simulink model "conSys_2robots_1_vR2014a"  (Simulink 8.3)
settings: Solver=FixedStepDiscrete  StartTime=0.0  StopTime=100  FixedStep=Ts  RelTol=1e-3
values from neighbouring files (symbols this model uses):
  ck = double(max(abs([par.q0_r1;par.q0_r2] - [par.q0r_r1;par.q0r_r2]))*20/7000 + 6)    [startUp_conSys_2robots_1_vGPU_vR2014a.m]    (also in startUp_conSys_2robots_1_vR2014a.m = max(abs([par.q0_r1;par.q0_r2] - [par.q0r_r1;par.q0r_r2]))*20; startUp_conSys_2robots_2_vR2014a.m = max(abs([par.q0_r1;par.q0_r2] - [par.q0r_r1;par.q0r_r2]))*20; startUp_conSys_2robots_3_vR2014a.m = max(abs([par.q0_r1;par.q0_r2] - [par.q0r_r1;par.q0r_r2]))*20; startUp_conSys_2robots_4_vR2014a.m = max(abs([par.q0_r1;par.q0_r2] - [par.q0r_r1;par.q0r_r2]))*20)
  d_0 = 2000    [startUp_conSys_2robots_1_vGPU_vR2014a.m]    (also in startUp_conSys_2robots_1_vR2014a.m = 200; startUp_conSys_2robots_2_vR2014a.m = 200; startUp_conSys_2robots_3_vR2014a.m; startUp_conSys_2robots_4_vR2014a.m = 200)
  do1r_0 = dthc_0 + dph1_0    (= 0.2)    [startUp_conSys_2robots_1_vGPU_vR2014a.m]    (also in startUp_conSys_2robots_1_vR2014a.m = 0; startUp_conSys_2robots_2_vR2014a.m = 0; startUp_conSys_2robots_3_vR2014a.m = 0; startUp_conSys_2robots_4_vR2014a.m = 0)
  do2r_0 = dthc_0 + dph2_0    (= -0.2)    [startUp_conSys_2robots_1_vGPU_vR2014a.m]    (also in startUp_conSys_2robots_1_vR2014a.m = 0; startUp_conSys_2robots_2_vR2014a.m = 0; startUp_conSys_2robots_3_vR2014a.m = 0; startUp_conSys_2robots_4_vR2014a.m = 0)
  dx1r_0 = dxc_0 + sin(thc_0)*dd_0 + d_0*cos(thc_0)*dthc_0    [startUp_conSys_2robots_1_vGPU_vR2014a.m]    (also in startUp_conSys_2robots_1_vR2014a.m; startUp_conSys_2robots_2_vR2014a.m; startUp_conSys_2robots_3_vR2014a.m; startUp_conSys_2robots_4_vR2014a.m)
  dx2r_0 = dxc_0 - sin(thc_0)*dd_0 - d_0*cos(thc_0)*dthc_0    [startUp_conSys_2robots_1_vGPU_vR2014a.m]    (also in startUp_conSys_2robots_1_vR2014a.m; startUp_conSys_2robots_2_vR2014a.m; startUp_conSys_2robots_3_vR2014a.m; startUp_conSys_2robots_4_vR2014a.m)
  dy1r_0 = dyc_0 + cos(thc_0)*dd_0 - d_0*sin(thc_0)*dthc_0    [startUp_conSys_2robots_1_vGPU_vR2014a.m]    (also in startUp_conSys_2robots_1_vR2014a.m; startUp_conSys_2robots_2_vR2014a.m; startUp_conSys_2robots_3_vR2014a.m; startUp_conSys_2robots_4_vR2014a.m)
  dy2r_0 = dyc_0 - cos(thc_0)*dd_0 + d_0*sin(thc_0)*dthc_0    [startUp_conSys_2robots_1_vGPU_vR2014a.m]    (also in startUp_conSys_2robots_1_vR2014a.m; startUp_conSys_2robots_2_vR2014a.m; startUp_conSys_2robots_3_vR2014a.m; startUp_conSys_2robots_4_vR2014a.m)
  o1r_0 = pi/2 - thc_0    (= 0)    [startUp_conSys_2robots_1_vGPU_vR2014a.m]    (also in startUp_conSys_2robots_1_vR2014a.m = pi/2 - thc_0; startUp_conSys_2robots_2_vR2014a.m = pi/2 - thc_0; startUp_conSys_2robots_3_vR2014a.m; startUp_conSys_2robots_4_vR2014a.m = th1_0)
  o2r_0 = pi/2 - thc_0    (= 0)    [startUp_conSys_2robots_1_vGPU_vR2014a.m]    (also in startUp_conSys_2robots_1_vR2014a.m = pi/2 - thc_0; startUp_conSys_2robots_2_vR2014a.m = pi/2 - thc_0; startUp_conSys_2robots_3_vR2014a.m; startUp_conSys_2robots_4_vR2014a.m = th2_0)
  thc_0 = pi/2    (= 1.57079632679)    [startUp_conSys_2robots_1_vGPU_vR2014a.m]    (also in startUp_conSys_2robots_1_vR2014a.m = atan2(1/25,1/12.5) + pi/2; startUp_conSys_2robots_2_vR2014a.m = atan2(1/25,1/12.5) + pi/2; startUp_conSys_2robots_3_vR2014a.m; startUp_conSys_2robots_4_vR2014a.m = atan2(1/25,1/12.5) + pi/2)
  Ts = 1/200    (= 0.005)    [startUp_conSys_2robots_1_vGPU_vR2014a.m]    (also in startUp_conSys_2robots_1_vR2014a.m = 0.0125; startUp_conSys_2robots_2_vR2014a.m = 0.01; startUp_conSys_2robots_3_vR2014a.m; startUp_conSys_2robots_4_vR2014a.m)
  x1_0 = 12000    [startUp_conSys_2robots_1_vGPU_vR2014a.m]    (also in startUp_conSys_2robots_1_vR2014a.m = 13178.9; startUp_conSys_2robots_2_vR2014a.m = 13178.9; startUp_conSys_2robots_3_vR2014a.m; startUp_conSys_2robots_4_vR2014a.m = 13178.9)
  x2_0 = 8000    [startUp_conSys_2robots_1_vGPU_vR2014a.m]    (also in startUp_conSys_2robots_1_vR2014a.m = 12821.1; startUp_conSys_2robots_2_vR2014a.m = 12821.1; startUp_conSys_2robots_3_vR2014a.m; startUp_conSys_2robots_4_vR2014a.m = 12821.1)
  xc_0 = 10000    [startUp_conSys_2robots_1_vGPU_vR2014a.m]    (also in startUp_conSys_2robots_1_vR2014a.m = 13000; startUp_conSys_2robots_2_vR2014a.m = 13000; startUp_conSys_2robots_3_vR2014a.m; startUp_conSys_2robots_4_vR2014a.m = 13000)
  y1_0 = 10000    [startUp_conSys_2robots_1_vGPU_vR2014a.m]    (also in startUp_conSys_2robots_1_vR2014a.m = 12910.6; startUp_conSys_2robots_2_vR2014a.m = 12910.6; startUp_conSys_2robots_3_vR2014a.m; startUp_conSys_2robots_4_vR2014a.m = 12910.6)
  y2_0 = 10000    [startUp_conSys_2robots_1_vGPU_vR2014a.m]    (also in startUp_conSys_2robots_1_vR2014a.m = 13089.4; startUp_conSys_2robots_2_vR2014a.m = 13089.4; startUp_conSys_2robots_3_vR2014a.m; startUp_conSys_2robots_4_vR2014a.m = 13089.4)
  yc_0 = 10000    [startUp_conSys_2robots_1_vGPU_vR2014a.m]    (also in startUp_conSys_2robots_1_vR2014a.m = 13000; startUp_conSys_2robots_2_vR2014a.m = 13000; startUp_conSys_2robots_3_vR2014a.m; startUp_conSys_2robots_4_vR2014a.m = 13000)
undefined symbols (not defined in the file or in its folder): absoluteAngle01_vR2014a, absoluteAngle02_vR2014a, DiscIntNeverNeededParam
undefined symbols (not defined in the file): ADAMS_cwd, ADAMS_exec, ADAMS_host, ADAMS_init, ADAMS_inputs, ADAMS_outputs, ADAMS_prefix, ADAMS_static, ADAMS_sysdir
libraries: simulink x18, cstblocks x7
(part 1 of 2)
settings Model: Creator=baqumau  LastModifiedBy=Mauro
settings DataIOCC: SignalLoggingSaveFormat=Dataset
settings DebuggingCC: UnderspecifiedInitializationDetection=Simplified  StateNameClashWarn=none
settings GRTTargetCC: CombineOutputUpdateFcns=on  GRTInterface=off

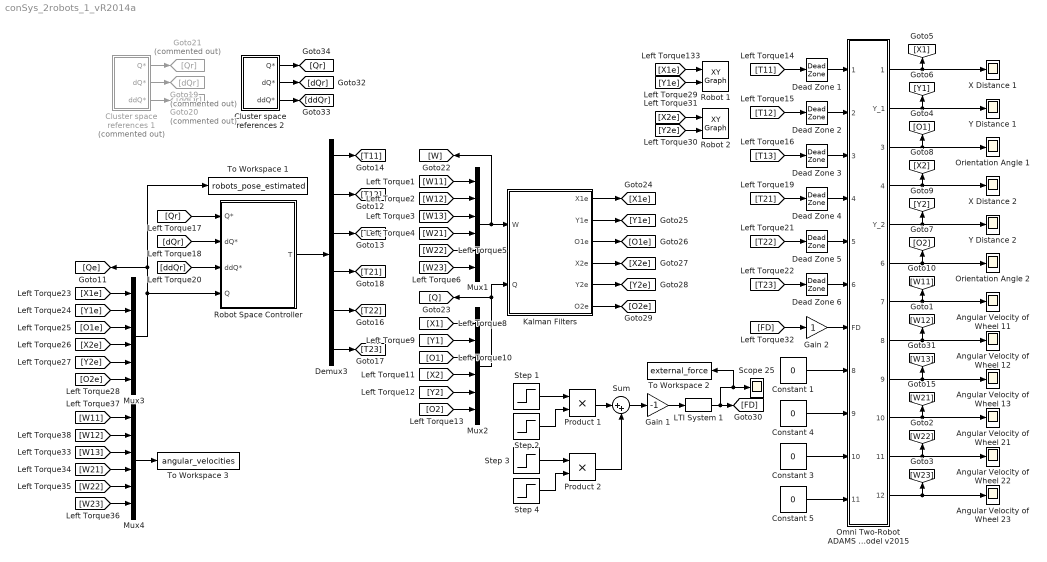
== system conSys_2robots_1_vR2014a ==
  Angular Velocity of Wheel {11..13,21..23} (6 alike) : Scope
      Angular Velocity of Wheel 11 settings: YMin=-1  YMax=20  SaveName=ScopeData3
      Angular Velocity of Wheel 12 settings: YMin=-1  YMax=20  SaveName=ScopeData6
      Angular Velocity of Wheel 13 settings: YMin=-1  YMax=1  SaveName=ScopeData9
      Angular Velocity of Wheel 21 settings: YMin=-1  YMax=1  SaveName=ScopeData2
      Angular Velocity of Wheel 22 settings: YMin=-1  YMax=1  SaveName=ScopeData10
      Angular Velocity of Wheel 23 settings: YMin=-1  YMax=1  SaveName=ScopeData11
  Cluster space references 1 : Subsystem  Commented=on
  Cluster space references 2 : Subsystem
  Constant {1,3..5} (4 alike) : Constant  Value=0
  Dead Zone {1..6} (6 alike) : DeadZone  LowerValue=-25  UpperValue=25  SaturateOnIntegerOverflow=on
  Demux3 : Demux  Outputs=6
  Gain 1 : Gain  Gain=-1
  Gain 2 : Gain
  Goto19 : Goto  Commented=on  GotoTag=dQr
  Goto20 : Goto  Commented=on  GotoTag=ddQr
  Goto21 : Goto  Commented=on  GotoTag=Qr
  Kalman Filters : Subsystem
  LTI System 1 : cstblocks/LTI System  sys=Fz  IC=[]
  Mux{1..4} (4 alike) : Mux  Inputs=6
  Omni Two-Robot ADAMS Model v2015 : Subsystem
  Orientation Angle 1 : Scope
      settings: YMin=-3  YMax=3
  Orientation Angle 2 : Scope
      settings: YMin=-3  YMax=3  SaveName=ScopeData12
  Product 1 : Product
  Product 2 : Product
  Robot 1 : simulink/Sinks/XY Graph  xmin=0  xmax=20000  ymin=0  ymax=20000  st=-1
  Robot 2 : simulink/Sinks/XY Graph  xmin=0  xmax=20000  ymin=0  ymax=20000  st=-1
  Robot Space Controller : Subsystem
  Scope 25 : Scope
      settings: YMin=-6  YMax=6  SaveName=ScopeData36
  Step 1 : Step  Time=60  SampleTime=0
  Step 2 : Step  Time=100  Before=1  After=0  SampleTime=0
  Step 3 : Step  Time=130  After=-1  SampleTime=0
  Step 4 : Step  Time=170  Before=1  After=0  SampleTime=0
  Sum : Sum  Inputs=|++
  To Workspace 1 : ToWorkspace  VariableName=robots_pose_estimated  SaveFormat=Structure With Time  SampleTime=-1
  To Workspace 2 : ToWorkspace  VariableName=external_force  SaveFormat=Structure With Time  SampleTime=-1
  To Workspace 3 : ToWorkspace  VariableName=angular_velocities  SaveFormat=Structure With Time  SampleTime=-1
  X Distance 1 : Scope
      settings: YMin=0  YMax=20000  SaveName=ScopeData4
  X Distance 2 : Scope
      settings: YMin=0  YMax=20000  SaveName=ScopeData16
  Y Distance 1 : Scope
      settings: YMin=0  YMax=20000
  Y Distance 2 : Scope
      settings: YMin=3000  YMax=3050  SaveName=ScopeData17
  wires:
  Omni Two-Robot ADAMS Model v2015/1(X_1) -> X Distance 1/1, [X1]
  Omni Two-Robot ADAMS Model v2015/2(Y_1) -> [Y1], Y Distance 1/1
  Omni Two-Robot ADAMS Model v2015/3(O_1) -> [O1], Orientation Angle 1/1
  Omni Two-Robot ADAMS Model v2015/7(W_11) -> [W11], Angular Velocity of Wheel 11/1
  Omni Two-Robot ADAMS Model v2015/10(W_21) -> [W21], Angular Velocity of Wheel 21/1
  Omni Two-Robot ADAMS Model v2015/9(W_13) -> Angular Velocity of Wheel 13/1, [W13]
  Omni Two-Robot ADAMS Model v2015/4(X_2) -> X Distance 2/1, [X2]
  Omni Two-Robot ADAMS Model v2015/5(Y_2) -> Y Distance 2/1, [Y2]
  Omni Two-Robot ADAMS Model v2015/6(O_2) -> Orientation Angle 2/1, [O2]
  Omni Two-Robot ADAMS Model v2015/8(W_12) -> Angular Velocity of Wheel 12/1, [W12]
  Omni Two-Robot ADAMS Model v2015/11(W_22) -> Angular Velocity of Wheel 22/1, [W22]
  Omni Two-Robot ADAMS Model v2015/12(W_23) -> [W23], Angular Velocity of Wheel 23/1
  [O1e] -> Mux3/3
  [X2e] -> Mux3/4
  [Y2e] -> Mux3/5
  [O2e] -> Mux3/6
  [X1e] -> Mux3/1
  [Y1e] -> Mux3/2
  [Qr] -> Robot Space Controller/1(Q*)
  [dQr] -> Robot Space Controller/2(dQ*)
  Mux3/1 -> Robot Space Controller/4(Q), [Qe], To Workspace 1/1
  Robot Space Controller/1(T) -> Demux3/1
  Demux3/1 -> [T11]
  Demux3/2 -> [T12]
  Demux3/3 -> [T13]
  Demux3/4 -> [T21]
  Demux3/5 -> [T22]
  Demux3/6 -> [T23]
  Cluster space references 1/1(Q*) -> Goto21/1
  Cluster space references 1/2(dQ*) -> Goto19/1
  Cluster space references 1/3(ddQ*) -> Goto20/1
  [ddQr] -> Robot Space Controller/3(ddQ*)
  [W13] -> Mux1/3
  [W21] -> Mux1/4
  [W22] -> Mux1/5
  [W23] -> Mux1/6
  [W11] -> Mux1/1
  [W12] -> Mux1/2
  Mux1/1 -> Kalman Filters/1(W), [W]
  [O1] -> Mux2/3
  [X2] -> Mux2/4
  [Y2] -> Mux2/5
  [O2] -> Mux2/6
  [X1] -> Mux2/1
  [Y1] -> Mux2/2
  Mux2/1 -> Kalman Filters/2(Q), [Q]
  Kalman Filters/1(X1e) -> [X1e]
  Kalman Filters/2(Y1e) -> [Y1e]
  Kalman Filters/3(O1e) -> [O1e]
  Kalman Filters/4(X2e) -> [X2e]
  Kalman Filters/5(Y2e) -> [Y2e]
  Kalman Filters/6(O2e) -> [O2e]
  [T11] -> Dead Zone 1/1
  [T12] -> Dead Zone 2/1
  [T13] -> Dead Zone 3/1
  [T21] -> Dead Zone 4/1
  [T22] -> Dead Zone 5/1
  [T23] -> Dead Zone 6/1
  [FD] -> Gain 2/1
  Constant 1/1 -> Omni Two-Robot ADAMS Model v2015/8(FX_1)
  Constant 3/1 -> Omni Two-Robot ADAMS Model v2015/10(FY_1)
  Constant 4/1 -> Omni Two-Robot ADAMS Model v2015/9(FX_2)
  Constant 5/1 -> Omni Two-Robot ADAMS Model v2015/11(FY_2)
  [X1e] -> Robot 1/1
  [Y1e] -> Robot 1/2
  [X2e] -> Robot 2/1
  [Y2e] -> Robot 2/2
  Step 1/1 -> Product 1/1
  Step 2/1 -> Product 1/2
  Step 3/1 -> Product 2/1
  Step 4/1 -> Product 2/2
  Product 1/1 -> Sum/1
  Product 2/1 -> Sum/2
  Sum/1 -> Gain 1/1
  LTI System 1/1 -> To Workspace 2/1, Scope 25/1, [FD]
  Gain 1/1 -> LTI System 1/1
  [W13] -> Mux4/3
  [W21] -> Mux4/4
  [W22] -> Mux4/5
  [W23] -> Mux4/6
  [W11] -> Mux4/1
  [W12] -> Mux4/2
  Mux4/1 -> To Workspace 3/1
  Gain 2/1 -> Omni Two-Robot ADAMS Model v2015/7(FD)
  Cluster space references 2/1(Q*) -> [Qr]
  Cluster space references 2/2(dQ*) -> [dQr]
  Cluster space references 2/3(ddQ*) -> [ddQr]
  Dead Zone 1/1 -> Omni Two-Robot ADAMS Model v2015/1(T_11)
  Dead Zone 2/1 -> Omni Two-Robot ADAMS Model v2015/2(T_12)
  Dead Zone 3/1 -> Omni Two-Robot ADAMS Model v2015/3(T_13)
  Dead Zone 4/1 -> Omni Two-Robot ADAMS Model v2015/4(T_21)
  Dead Zone 5/1 -> Omni Two-Robot ADAMS Model v2015/5(T_22)
  Dead Zone 6/1 -> Omni Two-Robot ADAMS Model v2015/6(T_23)

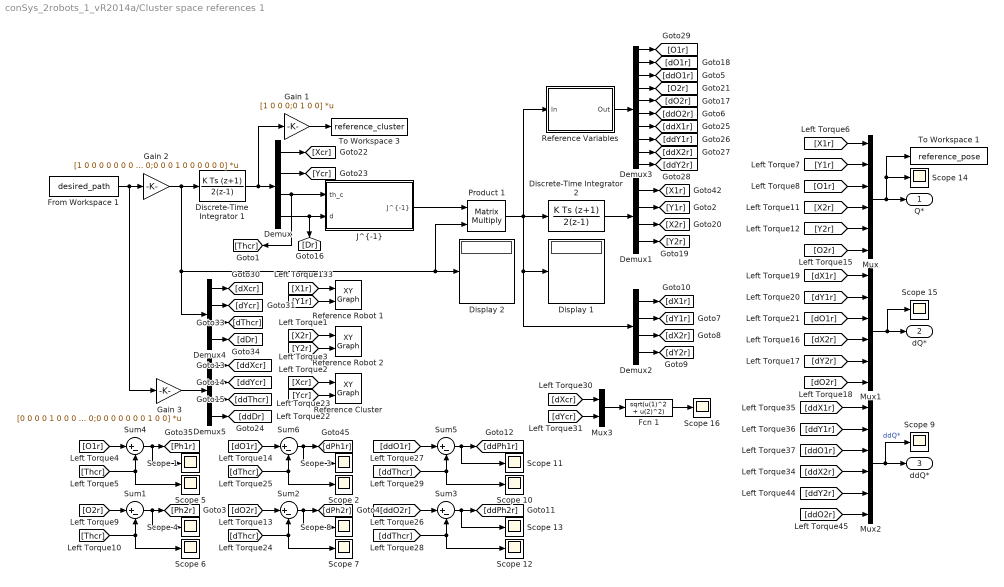
== system conSys_2robots_1_vR2014a/Cluster space references 1 ==
  Demux{,1..2,4..5} (5 alike) : Demux
  Demux3 : Demux  Outputs=10
  Discrete-Time Integrator 1 : DiscreteIntegrator  IntegratorMethod=Integration: Trapezoidal  InitialCondition=[xc_0 yc_0 thc_0 d_0]'  SampleTime=Ts  ICPrevOutput=DiscIntNeverNeededParam  ICPrevScaledInput=DiscIntNeverNeededParam
  Discrete-Time Integrator 2 : DiscreteIntegrator  IntegratorMethod=Integration: Trapezoidal  InitialCondition=[x1_0 y1_0 x2_0 y2_0]'  SampleTime=Ts  ICPrevOutput=DiscIntNeverNeededParam  ICPrevScaledInput=DiscIntNeverNeededParam
  Display 1 : Display
  Display 2 : Display
  Fcn 1 : Fcn  Expr=sqrt(u(1)^2 + u(2)^2)
  From Workspace 1 : FromWorkspace  VariableName=desired_path  SampleTime=Ts  OutputAfterFinalValue=Holding final value
  Gain 1 : Gain  Gain=[1 0 0 0;0 1 0 0]  Multiplication=Matrix(K*u)
  Gain 2 : Gain  Gain=[1 0 0 0 0 0 0 0 0 0;0 1 0 0 0 0 0 0 0 0;0 0 1 0 0 0 0 0 0 0;0 0 0 1 0 0 0 0 0 0]  Multiplication=Matrix(K*u)
  Gain 3 : Gain  Gain=[0 0 0 0 1 0 0 0 0 0;0 0 0 0 0 1 0 0 0 0;0 0 0 0 0 0 1 0 0 0;0 0 0 0 0 0 0 1 0 0]  Multiplication=Matrix(K*u)
  "J^{-1}" : Subsystem
  Mux : Mux  Inputs=6
  Mux1 : Mux  Inputs=6
  Mux2 : Mux  Inputs=6
  Mux3 : Mux  Inputs=2
  Product 1 : Product  Multiplication=Matrix(*)
  Reference Cluster : simulink/Sinks/XY Graph  xmin=0  xmax=20000  ymin=0  ymax=20000  st=-1
  Reference Robot 1 : simulink/Sinks/XY Graph  xmin=0  xmax=20000  ymin=0  ymax=20000  st=-1
  Reference Robot 2 : simulink/Sinks/XY Graph  xmin=0  xmax=20000  ymin=0  ymax=20000  st=-1
  Reference Variables : Subsystem
  Scope {1..16} (16 alike) : Scope
      Scope 1 settings: TimeRange=500  YMin=-15  YMax=15  SaveName=ScopeData52
      Scope 10 settings: TimeRange=500  YMin=-15  YMax=15  SaveName=ScopeData28
      Scope 11 settings: TimeRange=500  YMin=-15  YMax=15  SaveName=ScopeData42
      Scope 12 settings: TimeRange=500  YMin=-15  YMax=15  SaveName=ScopeData60
      Scope 13 settings: TimeRange=500  YMin=-15  YMax=15  SaveName=ScopeData66
      Scope 14 settings: ShowLegends=on  TimeRange=500  YMin=-6  YMax=0  SaveName=ScopeData59
      Scope 15 settings: ShowLegends=on  TimeRange=500  YMin=-1  YMax=1  SaveName=ScopeData69
      Scope 16 settings: ShowLegends=on  TimeRange=500  YMin=-50  YMax=200  SaveName=ScopeData18
      Scope 2 settings: TimeRange=500  YMin=-1  YMax=1  SaveName=ScopeData53
      Scope 3 settings: TimeRange=500  YMin=-1  YMax=1  SaveName=ScopeData79
      Scope 4 settings: TimeRange=500  YMin=-15  YMax=15  SaveName=ScopeData62
      Scope 5 settings: TimeRange=500  YMin=-15  YMax=15  SaveName=ScopeData81
      Scope 6 settings: TimeRange=500  YMin=-15  YMax=15  SaveName=ScopeData63
      Scope 7 settings: TimeRange=500  YMin=-15  YMax=15  SaveName=ScopeData64
      Scope 8 settings: TimeRange=500  YMin=-1  YMax=1  SaveName=ScopeData65
      Scope 9 settings: ShowLegends=on  TimeRange=500  YMin=-0.15  YMax=0.15  SaveName=ScopeData80
  Sum{1..6} (6 alike) : Sum  Inputs=|+-
  To Workspace 1 : ToWorkspace  VariableName=reference_pose  SaveFormat=Structure With Time  SampleTime=-1
  To Workspace 3 : ToWorkspace  VariableName=reference_cluster  SaveFormat=Structure With Time  SampleTime=-1
  Q* : Outport
  dQ* : Outport  Port=2
  ddQ* : Outport  Port=3
  wires:
  Demux4/1 -> [dXcr]
  Demux4/2 -> [dYcr]
  Demux4/4 -> [dDr]
  [Thcr] -> Scope 5/1, Sum4/2
  Demux4/3 -> [dThcr]
  Sum6/1 -> Scope 3/1, [dPh1r]
  Sum4/1 -> Scope 1/1, [Ph1r]
  [O1r] -> Sum4/1
  [dO1r] -> Sum6/1
  [dThcr] -> Scope 2/1, Sum6/2
  "J^{-1}"/1("J^{-1}") -> Product 1/1
  Product 1/1 -> Reference Variables/1(In), Demux2/1, Display 1/1, Discrete-Time Integrator 2/1
  [X1r] -> Reference Robot 1/1
  [Y1r] -> Reference Robot 1/2
  [X2r] -> Reference Robot 2/1
  [Y2r] -> Reference Robot 2/2
  From Workspace 1/1 -> Gain 3/1, Gain 2/1
  Discrete-Time Integrator 2/1 -> Demux1/1
  Demux1/1 -> [X1r]
  Demux1/2 -> [Y1r]
  Demux1/3 -> [X2r]
  Demux1/4 -> [Y2r]
  Reference Variables/1(Out) -> Demux3/1
  Demux3/1 -> [O1r]
  Demux3/2 -> [dO1r]
  Discrete-Time Integrator 1/1 -> Gain 1/1, Demux/1
  Demux/1 -> [Xcr]
  Demux/2 -> [Ycr]
  Demux/3 -> [Thcr], "J^{-1}"/1(th_c)
  Demux/4 -> [Dr], "J^{-1}"/2(d)
  Gain 1/1 -> To Workspace 3/1
  [X2r] -> Mux/4
  [O1r] -> Mux/3
  [Y1r] -> Mux/2
  [Y2r] -> Mux/5
  [X1r] -> Mux/1
  [O2r] -> Mux/6
  [dX2r] -> Mux1/4
  [dX1r] -> Mux1/1
  [dO1r] -> Mux1/3
  [dO2r] -> Mux1/6
  [dY2r] -> Mux1/5
  [dY1r] -> Mux1/2
  Mux/1 -> To Workspace 1/1, Scope 14/1, Q*/1
  Mux1/1 -> Scope 15/1, dQ*/1
  [Xcr] -> Reference Cluster/1
  [Ycr] -> Reference Cluster/2
  [Thcr] -> Sum1/2, Scope 6/1
  Sum1/1 -> [Ph2r], Scope 4/1
  [O2r] -> Sum1/1
  Sum2/1 -> [dPh2r], Scope 8/1
  [dO2r] -> Sum2/1
  [dThcr] -> Sum2/2, Scope 7/1
  Demux2/1 -> [dX1r]
  Demux2/2 -> [dY1r]
  Demux2/3 -> [dX2r]
  Demux2/4 -> [dY2r]
  Mux2/1 -> ddQ*/1, Scope 9/1  "ddQ*"
  [ddX1r] -> Mux2/1
  [ddY1r] -> Mux2/2
  [ddO1r] -> Mux2/3
  [ddX2r] -> Mux2/4
  [ddY2r] -> Mux2/5
  [ddO2r] -> Mux2/6
  Gain 2/1 -> Demux4/1, Product 1/2, Display 2/1, Discrete-Time Integrator 1/1
  Gain 3/1 -> Demux5/1
  Demux5/1 -> [ddXcr]
  Demux5/2 -> [ddYcr]
  Demux5/3 -> [ddThcr]
  Demux5/4 -> [ddDr]
  Demux3/4 -> [O2r]
  Demux3/5 -> [dO2r]
  Demux3/3 -> [ddO1r]
  Demux3/6 -> [ddO2r]
  Sum5/1 -> [ddPh1r], Scope 11/1
  [ddO1r] -> Sum5/1
  [ddThcr] -> Sum5/2, Scope 10/1
  Sum3/1 -> Scope 13/1, [ddPh2r]
  [ddO2r] -> Sum3/1
  [ddThcr] -> Scope 12/1, Sum3/2
  Demux3/7 -> [ddX1r]
  Demux3/8 -> [ddY1r]
  Demux3/9 -> [ddX2r]
  Demux3/10 -> [ddY2r]
  [dXcr] -> Mux3/1
  [dYcr] -> Mux3/2
  Mux3/1 -> Fcn 1/1
  Fcn 1/1 -> Scope 16/1

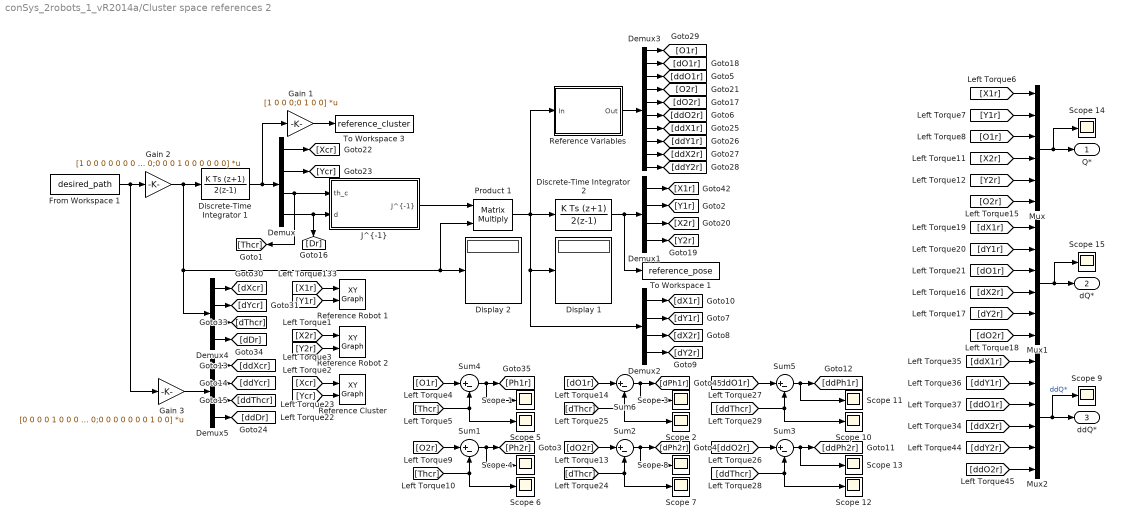
== system conSys_2robots_1_vR2014a/Cluster space references 2 ==
  Demux{,1..2,4..5} (5 alike) : Demux
  Demux3 : Demux  Outputs=10
  Discrete-Time Integrator 1 : DiscreteIntegrator  IntegratorMethod=Integration: Trapezoidal  InitialCondition=[xc_0 yc_0 thc_0 d_0]'  SampleTime=Ts  ICPrevOutput=DiscIntNeverNeededParam  ICPrevScaledInput=DiscIntNeverNeededParam
  Discrete-Time Integrator 2 : DiscreteIntegrator  IntegratorMethod=Integration: Trapezoidal  InitialCondition=[x1_0 y1_0 x2_0 y2_0]'  SampleTime=Ts  ICPrevOutput=DiscIntNeverNeededParam  ICPrevScaledInput=DiscIntNeverNeededParam
  Display 1 : Display
  Display 2 : Display
  From Workspace 1 : FromWorkspace  VariableName=desired_path  SampleTime=Ts  OutputAfterFinalValue=Holding final value
  Gain 1 : Gain  Gain=[1 0 0 0;0 1 0 0]  Multiplication=Matrix(K*u)
  Gain 2 : Gain  Gain=[1 0 0 0 0 0 0 0 0 0;0 1 0 0 0 0 0 0 0 0;0 0 1 0 0 0 0 0 0 0;0 0 0 1 0 0 0 0 0 0]  Multiplication=Matrix(K*u)
  Gain 3 : Gain  Gain=[0 0 0 0 1 0 0 0 0 0;0 0 0 0 0 1 0 0 0 0;0 0 0 0 0 0 1 0 0 0;0 0 0 0 0 0 0 1 0 0]  Multiplication=Matrix(K*u)
  "J^{-1}" : Subsystem
  Mux : Mux  Inputs=6
  Mux1 : Mux  Inputs=6
  Mux2 : Mux  Inputs=6
  Product 1 : Product  Multiplication=Matrix(*)
  Reference Cluster : simulink/Sinks/XY Graph  xmin=0  xmax=20000  ymin=0  ymax=20000  st=-1
  Reference Robot 1 : simulink/Sinks/XY Graph  xmin=0  xmax=20000  ymin=0  ymax=20000  st=-1
  Reference Robot 2 : simulink/Sinks/XY Graph  xmin=0  xmax=20000  ymin=0  ymax=20000  st=-1
  Reference Variables : Subsystem
  Scope {1..15} (15 alike) : Scope
      Scope 1 settings: TimeRange=500  YMin=-15  YMax=15  SaveName=ScopeData52
      Scope 10 settings: TimeRange=500  YMin=-15  YMax=15  SaveName=ScopeData28
      Scope 11 settings: TimeRange=500  YMin=-15  YMax=15  SaveName=ScopeData42
      Scope 12 settings: TimeRange=500  YMin=-15  YMax=15  SaveName=ScopeData60
      Scope 13 settings: TimeRange=500  YMin=-15  YMax=15  SaveName=ScopeData66
      Scope 14 settings: ShowLegends=on  TimeRange=500  YMin=-6  YMax=0  SaveName=ScopeData59
      Scope 15 settings: ShowLegends=on  TimeRange=500  YMin=-1  YMax=1  SaveName=ScopeData69
      Scope 2 settings: TimeRange=500  YMin=-15  YMax=15  SaveName=ScopeData53
      Scope 3 settings: TimeRange=500  YMin=-15  YMax=15  SaveName=ScopeData79
      Scope 4 settings: TimeRange=500  YMin=-15  YMax=15  SaveName=ScopeData62
      Scope 5 settings: TimeRange=500  YMin=-15  YMax=15  SaveName=ScopeData81
      Scope 6 settings: TimeRange=500  YMin=-15  YMax=15  SaveName=ScopeData63
      Scope 7 settings: TimeRange=500  YMin=-15  YMax=15  SaveName=ScopeData64
      Scope 8 settings: TimeRange=500  YMin=-15  YMax=15  SaveName=ScopeData65
      Scope 9 settings: ShowLegends=on  TimeRange=500  YMin=-0.15  YMax=0.15  SaveName=ScopeData80
  Sum{1..6} (6 alike) : Sum  Inputs=|+-
  To Workspace 1 : ToWorkspace  VariableName=reference_pose  SaveFormat=Structure With Time  SampleTime=-1
  To Workspace 3 : ToWorkspace  VariableName=reference_cluster  SaveFormat=Structure With Time  SampleTime=-1
  Q* : Outport
  dQ* : Outport  Port=2
  ddQ* : Outport  Port=3
  wires:
  Demux4/1 -> [dXcr]
  Demux4/2 -> [dYcr]
  Demux4/4 -> [dDr]
  [Thcr] -> Scope 5/1, Sum4/2
  Demux4/3 -> [dThcr]
  Sum6/1 -> Scope 3/1, [dPh1r]
  Sum4/1 -> Scope 1/1, [Ph1r]
  [O1r] -> Sum4/1
  [dO1r] -> Sum6/1
  [dThcr] -> Scope 2/1, Sum6/2
  "J^{-1}"/1("J^{-1}") -> Product 1/1
  Product 1/1 -> Reference Variables/1(In), Demux2/1, Display 1/1, Discrete-Time Integrator 2/1
  [X1r] -> Reference Robot 1/1
  [Y1r] -> Reference Robot 1/2
  [X2r] -> Reference Robot 2/1
  [Y2r] -> Reference Robot 2/2
  From Workspace 1/1 -> Gain 3/1, Gain 2/1
  Discrete-Time Integrator 2/1 -> To Workspace 1/1, Demux1/1
  Demux1/1 -> [X1r]
  Demux1/2 -> [Y1r]
  Demux1/3 -> [X2r]
  Demux1/4 -> [Y2r]
  Discrete-Time Integrator 1/1 -> Gain 1/1, Demux/1
  Demux/1 -> [Xcr]
  Demux/2 -> [Ycr]
  Demux/3 -> [Thcr], "J^{-1}"/1(th_c)
  Demux/4 -> [Dr], "J^{-1}"/2(d)
  Gain 1/1 -> To Workspace 3/1
  [X2r] -> Mux/4
  [O1r] -> Mux/3
  [Y1r] -> Mux/2
  [Y2r] -> Mux/5
  [X1r] -> Mux/1
  [O2r] -> Mux/6
  [dX2r] -> Mux1/4
  [dX1r] -> Mux1/1
  [dO1r] -> Mux1/3
  [dO2r] -> Mux1/6
  [dY2r] -> Mux1/5
  [dY1r] -> Mux1/2
  Mux/1 -> Scope 14/1, Q*/1
  Mux1/1 -> Scope 15/1, dQ*/1
  [Xcr] -> Reference Cluster/1
  [Ycr] -> Reference Cluster/2
  [Thcr] -> Sum1/2, Scope 6/1
  Sum1/1 -> [Ph2r], Scope 4/1
  [O2r] -> Sum1/1
  Sum2/1 -> [dPh2r], Scope 8/1
  [dO2r] -> Sum2/1
  [dThcr] -> Sum2/2, Scope 7/1
  Demux2/1 -> [dX1r]
  Demux2/2 -> [dY1r]
  Demux2/3 -> [dX2r]
  Demux2/4 -> [dY2r]
  Mux2/1 -> ddQ*/1, Scope 9/1  "ddQ*"
  [ddX1r] -> Mux2/1
  [ddY1r] -> Mux2/2
  [ddO1r] -> Mux2/3
  [ddX2r] -> Mux2/4
  [ddY2r] -> Mux2/5
  [ddO2r] -> Mux2/6
  Gain 2/1 -> Demux4/1, Product 1/2, Display 2/1, Discrete-Time Integrator 1/1
  Gain 3/1 -> Demux5/1
  Demux5/1 -> [ddXcr]
  Demux5/2 -> [ddYcr]
  Demux5/3 -> [ddThcr]
  Demux5/4 -> [ddDr]
  Sum5/1 -> [ddPh1r], Scope 11/1
  [ddO1r] -> Sum5/1
  [ddThcr] -> Sum5/2, Scope 10/1
  Sum3/1 -> Scope 13/1, [ddPh2r]
  [ddO2r] -> Sum3/1
  [ddThcr] -> Scope 12/1, Sum3/2
  Reference Variables/1(Out) -> Demux3/1
  Demux3/1 -> [O1r]
  Demux3/2 -> [dO1r]
  Demux3/4 -> [O2r]
  Demux3/5 -> [dO2r]
  Demux3/3 -> [ddO1r]
  Demux3/6 -> [ddO2r]
  Demux3/7 -> [ddX1r]
  Demux3/8 -> [ddY1r]
  Demux3/9 -> [ddX2r]
  Demux3/10 -> [ddY2r]

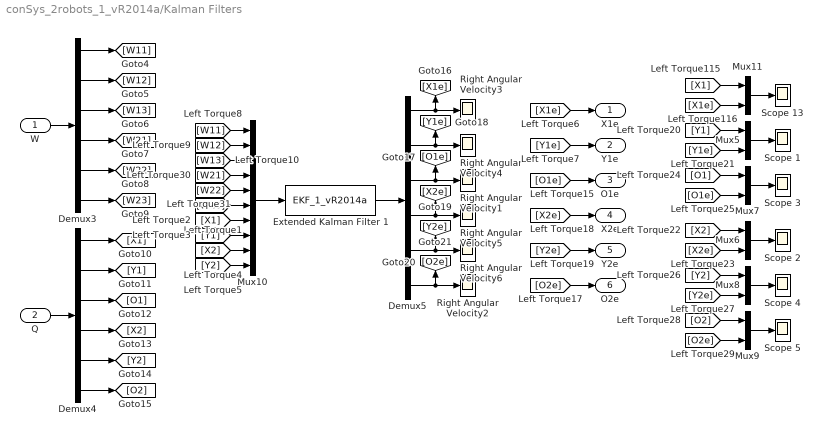
== system conSys_2robots_1_vR2014a/Kalman Filters ==
  W : Inport
  Q : Inport  Port=2
  Demux3 : Demux  Outputs=6
  Demux4 : Demux  Outputs=6
  Demux5 : Demux  Outputs=6
  Extended Kalman Filter 1 : S-Function  FunctionName=EKF_1_vR2014a  Parameters=par  EnableBusSupport=off
  Mux10 : Mux  Inputs=10
  Mux{5..9,11} (6 alike) : Mux  Inputs=2
  Right Angular Velocity{1..6} (6 alike) : Scope
      Right Angular Velocity1 settings: YMin=-3  YMax=6  SaveName=ScopeData5
      Right Angular Velocity2 settings: YMin=-3  YMax=6  SaveName=ScopeData13
      Right Angular Velocity3 settings: YMin=-10000  YMax=10000  SaveName=ScopeData7
      Right Angular Velocity4 settings: YMin=0  YMax=5000  SaveName=ScopeData8
      Right Angular Velocity5 settings: YMin=-10000  YMax=10000  SaveName=ScopeData14
      Right Angular Velocity6 settings: YMin=0  YMax=5000  SaveName=ScopeData15
  Scope {1..5,13} (6 alike) : Scope
      Scope 1 settings: YMin=0  YMax=20000  SaveName=ScopeData29
      Scope 13 settings: YMin=0  YMax=20000  SaveName=ScopeData25
      Scope 2 settings: YMin=-2  YMax=20000  SaveName=ScopeData32
      Scope 3 settings: YMin=-2  YMax=20  SaveName=ScopeData33
      Scope 4 settings: YMin=-2  YMax=20000  SaveName=ScopeData34
      Scope 5 settings: YMin=-2  YMax=20  SaveName=ScopeData35
  X1e : Outport
  Y1e : Outport  Port=2
  O1e : Outport  Port=3
  X2e : Outport  Port=4
  Y2e : Outport  Port=5
  O2e : Outport  Port=6
  wires:
  W/1 -> Demux3/1
  Demux3/1 -> [W11]
  Demux3/2 -> [W12]
  Demux3/3 -> [W13]
  Demux3/4 -> [W21]
  Demux3/5 -> [W22]
  Demux3/6 -> [W23]
  Demux4/1 -> [X1]
  Demux4/2 -> [Y1]
  Demux4/3 -> [O1]
  Demux4/4 -> [X2]
  Demux4/5 -> [Y2]
  Demux4/6 -> [O2]
  Q/1 -> Demux4/1
  [X1e] -> X1e/1
  [Y1e] -> Y1e/1
  [O1e] -> O1e/1
  [X2e] -> X2e/1
  [Y2e] -> Y2e/1
  [O2e] -> O2e/1
  [X1e] -> Mux11/2
  Mux11/1 -> Scope 13/1
  [X1] -> Mux11/1
  [Y1e] -> Mux5/2
  Mux5/1 -> Scope 1/1
  [Y1] -> Mux5/1
  [X2e] -> Mux6/2
  Mux6/1 -> Scope 2/1
  [X2] -> Mux6/1
  [O1e] -> Mux7/2
  Mux7/1 -> Scope 3/1
  [O1] -> Mux7/1
  [Y2e] -> Mux8/2
  Mux8/1 -> Scope 4/1
  [Y2] -> Mux8/1
  [O2e] -> Mux9/2
  Mux9/1 -> Scope 5/1
  [O2] -> Mux9/1
  [W11] -> Mux10/1
  [W12] -> Mux10/2
  [W13] -> Mux10/3
  Mux10/1 -> Extended Kalman Filter 1/1
  Extended Kalman Filter 1/1 -> Demux5/1
  Demux5/2 -> Right Angular Velocity4/1, [Y1e]
  Demux5/3 -> Right Angular Velocity1/1, [O1e]
  Demux5/1 -> Right Angular Velocity3/1, [X1e]
  [W21] -> Mux10/4
  [W22] -> Mux10/5
  Demux5/5 -> [Y2e], Right Angular Velocity6/1
  Demux5/6 -> [O2e], Right Angular Velocity2/1
  Demux5/4 -> [X2e], Right Angular Velocity5/1
  [W23] -> Mux10/6
  [X1] -> Mux10/7
  [Y1] -> Mux10/8
  [Y2] -> Mux10/10
  [X2] -> Mux10/9

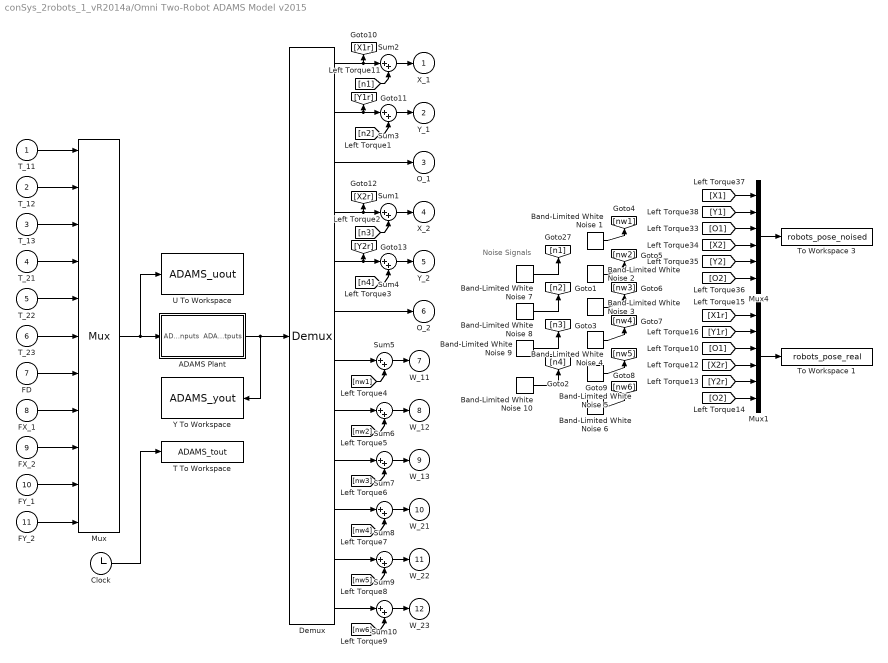
== system conSys_2robots_1_vR2014a/Omni Two-Robot ADAMS Model v2015 ==
  note: Noise Signals
  T_11 : Inport
  T_12 : Inport  Port=2
  T_13 : Inport  Port=3
  T_21 : Inport  Port=4
  T_22 : Inport  Port=5
  T_23 : Inport  Port=6
  FD : Inport  Port=7
  FX_1 : Inport  Port=8
  FX_2 : Inport  Port=9
  FY_1 : Inport  Port=10
  FY_2 : Inport  Port=11
  ADAMS Plant : Subsystem  LoadFcn=|  InitFcn=clear mex  mask(Adams Plant){exevie=ADAMS_sysdir, nam_in=ADAMS_inputs, namout=ADAMS_outputs, nampre=ADAMS_prefix, outfil=ADAMS_prefix, exesol=ADAMS_exec, stat=ADAMS_static, inicmd=[ADAMS_init], exetyp=C++, comtyp=PIPE(DDE), workdir=ADAMS_cwd, ada_host=ADAMS_host, modani=batch, modsim=discrete, dft=no, simulink_lead_cosim=yes, pin_interp_order=0, pout_extrap_order=0, pin_extrap_order=0, pout_interp_order=0, dt_out=Ts, o_rate=1, more=off}
      | %check based on dialog box setting for when setting by popup menu                                             
      | if exist('ADAMS_solver_type')                                                                                 
      |   if strcmp(ADAMS_solver_type,'C++')                                                                          
      |     set_param(gcb,'exetyp','C++');                                                                            
      |   else                                                                                                        
      |     set_param(gcb,'exetyp','Fortran');                                                                        
      |   end                                                                                                         
      | else                                                                                                          
      |   set_param(gcb,'exetyp','C++');                                                                              
      | end                                                                                                           
      | %set the mode if using acar_solver                                                                            
      | %REQUIRED HERE BECAUSE BELOW CAUSES MDLTERMINATE TO BE CALLED 2 TIMES IN MIDDLE OF SIMULATION WHEN SET IN MASK
      |                                                                                                               
      | %enable the direct feedthrough, sim mode, anim mode parameters by default                                     
      |                                                                                                               
      | if exist('set_some_params_states')                                                                            
      |                                                                                                               
      |   set_some_params_states({'dft','modsim','modani'},{'on','on','on'},'MaskEnables',gcb)                        
      |   %turn on direct feedthrough option                                                                          
      |   set_some_params_states({'dft'},{'on'},'MaskVisibilities',gcb)                                               
      |                                                                                                               
      |  end                                                                                                          
      |                                                                                                               
      |                                                                                                               
      | if exist('ADAMS_exec')                                                                                        
      |   if and(strcmp(get_param(gcb,'exesol'),'ADAMS_exec'),strcmp(ADAMS_exec,'acar_solver'))                       
      |     %set the sim mode to discrete -- only supported mode                                                      
      |     set_param(gcb,'modsim','discrete')                                                                        
      |      %turn off direct feedthrough option                                                                      
      |      set_some_params_states({'dft'},{'off'},'MaskVisibilities',gcb)                                           
      |     %set the animation mode to batch -- only supported mode                                                   
      |     set_param(gcb,'modani','batch')                                                                           
      |     %disable the direct feedthrough, sim mode, anim mode parameters                                           
      |     set_some_params_states({'modsim','modani'},{'off','off'},'MaskEnables',gcb)                               
      |   end                                                                                                         
      | end
      mask prompts: exevie "Adams install directory"; nam_in "Adams/View input names"; namout "Adams/View output names"; nampre "Adams model file prefix"; outfil "Output files prefix (opt.: if blank - no output)"; exesol "User executable (opt.: if blank - use standard)"; stat "Initial static simulation flag"; inicmd "Initialization commands"; exetyp "Adams/Solver type"; comtyp "Interprocess option"; workdir "Adams working directory"; ada_host "Adams host"; modani "Animation mode"; modsim "Simulation mode"; dft "Direct feedthrough"; simulink_lead_cosim "Discrete Computational Order - Simulink Leads Adams"; pin_interp_order "Plant input interpolation order"; pout_extrap_order "Plant output extrapolation order"; pin_extrap_order "Plant input extrapolation order"; pout_interp_order "Plant output interpolation order"; dt_out "Communication interval"; o_rate "Number of communications per output step"; more "More parameters"
      mask help: Simulate any Adams plant model either in Adams/Solver form (.adm file) or in Adams/View form (.cmd file)
      settings: OpenFcn=|
      | open_system(gcb,'mask')
      | if not(exist('set_some_params_states'))
      | 
      | warning('The script "set_some_params_states.m" cannot be found in the MATLAB PATH.  Cannot update the ADAMS Plant S-Function parameters.')
      | 
      | warning('Recommended action(optional):  run the Adams/Controls .m file first to help choose the correct settings in the Adams S-Function block.')
      | 
      | end
      mask Help:
      | <html>
      | This S-Function represents the non-linear Adams Plant with the inputs sent to the Adams model <br>
      |  and the outputs generated by the Adams model.  See the Adams/Controls documentation for more <br>
      | information.  This plant uses the following variables:<br>
      | <br>
      | <b>ADAMS_sysdir  :</b> Adams installation directory<br>
      | <b>ADAMS_inputs  :</b> Input variables View names vector<br>
      | <b>ADAMS_outputs :</b> Outputs variables View names vector<br>
      | <b>ADAMS_prefix  : </b>ADAMS model files prefix (.adm, .cmd); also doubles as output files prefix<br>
      | <b>ADAMS_exec :</b> Adams/Solver user library or keyword (e.g., acar_solver)<br>
      | <b>ADAMS_static :</b> yes|no - initial static before Co-simulation(discrete)/Function Evaluation(continuous)<br>
      | <b>ADAMS_init :</b>Initialization commands (i.e., Adams/View or Solver commands, depending on setting for Animation mode)<br>
      | <b>ADAMS_cwd : </b> Current working directory (for TCP/IP)<br>
      | <b>ADAMS_host : </b>Name of Adams server host (for TCP/IP)<br>
      | <b>ADAMS_mode :</b> Linear or non-linear (i.e., co-sim, function eval)<br>
      | <b>ADAMS_solver_type :</b>Fortran or C++ (used to set popup menu when first loaded) <br>
      | 
      | 
      | <br>
      | The following settings can be chosen:<br>
      | <br>
      | <b>Adams/Solver type:</b>  Fortran or C++ (will also set ADAMS_solver_type)<br>
      | <b>Interprocess option:</b> Pipe(DDE) or TCP/IP; TCP/IP can allow different machines run Adams and MATLAB<br>
      | <b>Animation mode:</b> batch (Solver, uses .adm) or interactive (View, uses .cmd)<br>
      | <b>Simulation mode:</b> discrete (Co-simulation) or continuous (Function Evaluation)<br>
      | <b>Discrete Computational Order - Simulink Lead Adams:</b> for discrete mode, chooses if Simulink leads the integration (yes) or lags (no);<br> if set to "no", can remove algebraic loop<br>
      | <b>Plant input interpolation order:</b> 0 = zero-order hold; 1 = linear (discrete mode only, where Simulink leads)<br>
      | <b>Plant output extrapolation order:</b> 0 = zero-order hold;1 = linear(discrete mode only, where Simulink leads)<br>
      | <b>Plant input extrapolation order:</b> 0 = zero-order hold; 1 = linear (discrete mode only, where Adams leads)<br>
      | <b>Plant output interpolation order:</b> 0 = zero-order hold;1 = linear(discrete mode only, where Adams leads)<br>
      | <b>Direct feedthrough:</b> yes|no - yes = Input directly effect output(continuous mode-only)<br>
      | <b>Communication interval:</b> Time step at which Co-simulation exchange information (e.g.,0.005); also controls <br>output for continuous mode (Function Evaluation)<br>
      | <b>Number of communications per output step: </b>Sets Adams output rate (.res, .req, .gra) integer value (default: 1)<br>
      | </html>
      mask Callback exesol:
      | if exist('set_some_params_states')
      | %enable the direct feedthrough, sim mode, anim mode parameters
      | set_some_params_states({'dft','modsim','modani'},{'on','on','on'},'MaskEnables',gcb)
      | %turn on direct feedthrough option
      | set_some_params_states({'dft'},{'on'},'MaskVisibilities',gcb)
      | end
      | 
      | if exist('ADAMS_exec')
      |   if and(strcmp(get_param(gcb,'exesol'),'ADAMS_exec'),strcmp(ADAMS_exec,'acar_solver'))
      |     %set the sim mode to discrete -- only supported mode
      |     %REMOVED:  BELOW CAUSES MDLTERMINATE TO BE CALLED 2 TIMES IN MIDDLE OF SIMULATION
      |     %Now in LoadFcn callback
      |     %set_param(gcb,'modsim','discrete')
      |      %turn off direct feedthrough option
      |     set_some_params_states({'dft'},{'off'},'MaskVisibilities',gcb)
      |     %set the animation mode to batch -- only supported mode
      |     %REMOVED:  BELOW CAUSES MDLTERMINATE TO BE CALLED 2 TIMES IN MIDDLE OF SIMULATION
      |     %Now in LoadFcn callback
      |     %set_param(gcb,'modani','batch')
      |     %disable the direct feedthrough, sim mode, anim mode parameters
      |     set_some_params_states({'modsim','modani'},{'off','off'},'MaskEnables',gcb)
      |   end
      | end
      mask TypeOptions exetyp: Fortran | C++
      mask Callback exetyp:
      | if strcmp(get_param(gcb,'exetyp'),'C++')
      |     ADAMS_solver_type='C++';
      | else
      |     ADAMS_solver_type='Fortran';
      | end
      mask TypeOptions comtyp: PIPE(DDE) | TCP/IP
      mask Callback comtyp:
      | if exist('set_some_params_states')
      | if strcmp(get_param(gcb,'comtyp'),'PIPE(DDE)')
      |     %turn off cwd, host options
      |     set_some_params_states({'ada_host','workdir'},{'off','off'},'MaskVisibilities',gcb)
      | else%if strcmp(get_param(gcb,'modsim'),'TCP/IP')
      |     %turn on cwd, host options
      |     set_some_params_states({'ada_host','workdir'},{'on','on'},'MaskVisibilities',gcb)
      | end
      | end
      mask TypeOptions modani: batch | interactive
      mask TypeOptions modsim: discrete | continuous
      mask Callback modsim:
      | if exist('set_some_params_states')
      | if strcmp(get_param(gcb,'modsim'),'discrete')
      |      %turn off direct feedthrough option
      |     set_some_params_states({'dft'},{'off'},'MaskVisibilities',gcb)
      |     %turn on discrete co-sim type if want to see more
      |     if strcmp(get_param(gcb,'more'),'on')
      |         set_some_params_states({'simulink_lead_cosim'},{'on'},'MaskVisibilities',gcb)
      |     end
      |     if strcmp(get_param(gcb,'simulink_lead_cosim'),'yes')
      |         %turn on interpolation/extrapolation options
      |         set_some_params_states({'pin_interp_order','pout_extrap_order',},{'on','on'},'MaskVisibilities',gcb)
      |     else
      |         set_some_params_states({'pin_extrap_order','pout_interp_order'},{'on','on'},'MaskVisibilities',gcb)
      |     end
      | else%if strcmp(get_param(gcb,'modsim'),'continuous')
      |      %turn off direct feedthrough option
      |     set_some_params_states({'dft'},{'on'},'MaskVisibilities',gcb)
      |     %turn off interpolation/extrapolation options
      |     set_some_params_states({'pin_interp_order','pout_extrap_order','pin_extrap_order','pout_interp_order','simulink_lead_cosim'},{'off','off','off','off','off'},'MaskVisibilities',gcb)
      | end
      | end
      mask TypeOptions dft: no | yes
      mask TypeOptions simulink_lead_cosim: yes | no
      mask Callback simulink_lead_cosim:
      | if exist('set_some_params_states')
      | if (strcmp(get_param(gcb,'simulink_lead_cosim'),'yes') && strcmp(get_param(gcb,'modsim'),'discrete'))
      |      %turn off unused interpolate/extrapolate options
      |     set_some_params_states({'pin_extrap_order','pout_interp_order'},{'off','off'},'MaskVisibilities',gcb)
      |     %turn on used interpolate/extrapolate options
      |     set_some_params_states({'pin_interp_order','pout_extrap_order'},{'on','on'},'MaskVisibilities',gcb)
      | elseif (strcmp(get_param(gcb,'simulink_lead_cosim'),'no') && strcmp(get_param(gcb,'modsim'),'discrete'))
      |     %turn on used interpolate/extrapolate options
      |     set_some_params_states({'pin_extrap_order','pout_interp_order'},{'on','on'},'MaskVisibilities',gcb)
      |      %turn off unused interpolate/extrapolate options
      |     set_some_params_states({'pin_interp_order','pout_extrap_order'},{'off','off'},'MaskVisibilities',gcb)
      | end
      | end
      mask TypeOptions pin_interp_order: 0 | 1
      mask TypeOptions pout_extrap_order: 0 | 1
      mask TypeOptions pin_extrap_order: 0 | 1
      mask TypeOptions pout_interp_order: 0 | 1
      mask Callback more:
      | if exist('set_some_params_states')
      | if (strcmp(get_param(gcb,'more'),'on'))
      |      %turn on infrequently used options
      |     set_some_params_states({'exevie','nam_in','namout','exesol','stat','inicmd'},{'on','on','on','on','on','on'},'MaskVisibilities',gcb)
      |     if strcmp(get_param(gcb,'modsim'),'discrete')
      |         set_some_params_states({'simulink_lead_cosim'},{'on'},'MaskVisibilities',gcb)
      |     end
      | elseif (strcmp(get_param(gcb,'more'),'off'))
      |     %turn off infrequently used options
      |     set_some_params_states({'exevie','nam_in','namout','exesol','stat','inicmd'},{'off','off','off','off','off','off'},'MaskVisibilities',gcb)
      |     if strcmp(get_param(gcb,'modsim'),'discrete')
      |         set_some_params_states({'simulink_lead_cosim'},{'off'},'MaskVisibilities',gcb)
      |     end
      | end
      | end
      mask Display: disp( 'MSC Software' )
  Band-Limited White Noise {1..6} (6 alike) : simulink/Sources/Band-Limited White Noise  Cov=[0.001]  Ts=Ts  seed=[23341]
  Band-Limited White Noise {7..10} (4 alike) : simulink/Sources/Band-Limited White Noise  Cov=[0.5]  Ts=Ts  seed=[23341]
  Clock : Clock
  Demux : Demux  Outputs=12
  Mux : Mux  Inputs=11
  Mux1 : Mux  Inputs=6
  Mux4 : Mux  Inputs=6
  Sum{1..10} (10 alike) : Sum  Inputs=|++
  T To Workspace : ToWorkspace  VariableName=ADAMS_tout
      settings: MaxDataPoints=100000
  To Workspace 1 : ToWorkspace  VariableName=robots_pose_real  SaveFormat=Structure With Time  SampleTime=-1
  To Workspace 3 : ToWorkspace  VariableName=robots_pose_noised  SaveFormat=Structure With Time  SampleTime=-1
  U To Workspace : ToWorkspace  VariableName=ADAMS_uout
      settings: MaxDataPoints=100000
  Y To Workspace : ToWorkspace  VariableName=ADAMS_yout
      settings: MaxDataPoints=100000
  X_1 : Outport
  Y_1 : Outport  Port=2
  O_1 : Outport  Port=3
  X_2 : Outport  Port=4
  Y_2 : Outport  Port=5
  O_2 : Outport  Port=6
  W_11 : Outport  Port=7
  W_12 : Outport  Port=8
  W_13 : Outport  Port=9
  W_21 : Outport  Port=10
  W_22 : Outport  Port=11
  W_23 : Outport  Port=12
  wires:
  FY_2/1 -> Mux/11
  FY_1/1 -> Mux/10
  FX_2/1 -> Mux/9
  FX_1/1 -> Mux/8
  FD/1 -> Mux/7
  T_23/1 -> Mux/6
  T_22/1 -> Mux/5
  T_21/1 -> Mux/4
  T_13/1 -> Mux/3
  T_12/1 -> Mux/2
  T_11/1 -> Mux/1
  Demux/1 -> [X1r], Sum2/1
  Demux/2 -> [Y1r], Sum3/1
  Sum2/1 -> X_1/1
  Sum3/1 -> Y_1/1
  Demux/4 -> [X2r], Sum1/1
  Demux/5 -> [Y2r], Sum4/1
  Sum1/1 -> X_2/1
  Sum4/1 -> Y_2/1
  [n1] -> Sum2/2
  [n2] -> Sum3/2
  [n3] -> Sum1/2
  [n4] -> Sum4/2
  [nw1] -> Sum5/2
  [nw2] -> Sum6/2
  [nw3] -> Sum7/2
  [nw4] -> Sum8/2
  [nw5] -> Sum9/2
  [nw6] -> Sum10/2
  Demux/7 -> Sum5/1
  Sum5/1 -> W_11/1
  Demux/8 -> Sum6/1
  Sum6/1 -> W_12/1
  Demux/9 -> Sum7/1
  Sum7/1 -> W_13/1
  Demux/10 -> Sum8/1
  Sum8/1 -> W_21/1
  Demux/11 -> Sum9/1
  Sum9/1 -> W_22/1
  Demux/12 -> Sum10/1
  Sum10/1 -> W_23/1
  Demux/3 -> O_1/1
  Demux/6 -> O_2/1
  Band-Limited White Noise 7/1 -> [n1]
  Band-Limited White Noise 8/1 -> [n2]
  Band-Limited White Noise 9/1 -> [n3]
  Band-Limited White Noise 10/1 -> [n4]
  Band-Limited White Noise 1/1 -> [nw1]
  Band-Limited White Noise 2/1 -> [nw2]
  Band-Limited White Noise 3/1 -> [nw3]
  Band-Limited White Noise 4/1 -> [nw4]
  Band-Limited White Noise 5/1 -> [nw5]
  Band-Limited White Noise 6/1 -> [nw6]
  [O1] -> Mux4/3
  [X2] -> Mux4/4
  [Y2] -> Mux4/5
  [O2] -> Mux4/6
  [X1] -> Mux4/1
  [Y1] -> Mux4/2
  Mux4/1 -> To Workspace 3/1
  [O1] -> Mux1/3
  [X2r] -> Mux1/4
  [Y2r] -> Mux1/5
  [O2] -> Mux1/6
  [X1r] -> Mux1/1
  [Y1r] -> Mux1/2
  Mux1/1 -> To Workspace 1/1
  Clock/1 -> T To Workspace/1
  Mux/1 -> U To Workspace/1, ADAMS Plant/1(ADAMS inputs)
  ADAMS Plant/1(ADAMS outputs) -> Y To Workspace/1, Demux/1
